simulink library "sm_excv_underc_lib"  (R2023b)
settings: Solver=VariableStepAuto  StartTime=0.0  StopTime=10.0  RelTol=1e-3
undefined symbols (not defined in the file): Excv, L1, L2, L3, L4, L5, L6, L7, L8, L9, P1, P2, P3, P4, P5, P6, P7, P8, P9, shoe_w, X, Y, Z
libraries: sm_tracked_vehicle_lib x70, sm_lib x54, nesl_utility x32, sm_excv_scene_lib x9, fl_lib x8, sm_excv_frame_lib x4
(part 2 of 5)

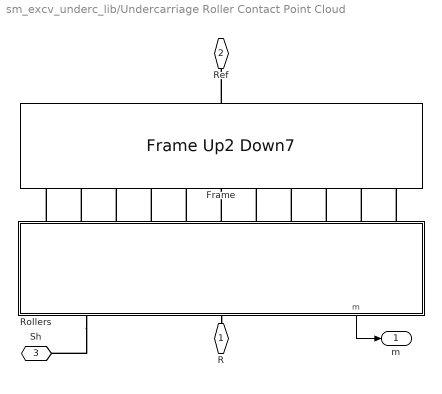
== system sm_excv_underc_lib/Undercarriage Roller Contact Point Cloud ==
  Frame : sm_excv_frame_lib/Frame Up2 Down7  roller_upper_x=roller_upper_x  roller_lower_x=roller_lower_x  idler_x=idler_x  roller_upper_y=roller_upper_y  sprk_pitch_rad=sprk_pitch_rad  roller_lower_rad=roller_lower_rad  plate_h=plate_h  idler_rad=idler_rad  idler_lower_roller_offset_y=idler_lower_roller_offset_y
  Rollers : Subsystem  mask(Rollers with Ground Contact (Point Cloud)){sprk_xc=sprk_xc, sprk_len=sprk_len, sprk_rho=sprk_rho, sprk_clr=sprk_clr, sprk_opc=sprk_opc, sprk_contact_geo_ptcld=sprk_contact_geo_ptcld, sprk_contact_geo_rad=sprk_contact_geo_rad, sprk_contact_geo_clr=sprk_contact_geo_clr, sprk_contact_geo_opc=sprk_contact_geo_opc, idler_rad=idler_rad, idler_len=idler_len, idler_rho=idler_rho, idler_clr=idler_clr, idler_opc=idler_opc, idler_contact_geo_ptcld=idler_contact_geo_ptcld, idler_contact_geo_rad=idler_contact_geo_rad, idler_contact_geo_clr=idler_contact_geo_clr, idler_contact_geo_opc=idler_contact_geo_opc, roller_upper_len=roller_upper_len, roller_upper_rad=roller_upper_rad, roller_upper_rho=roller_upper_rho, roller_upper_clr=roller_upper_clr, roller_upper_opc=roller_upper_opc, roller_upper_contgeo_clr=roller_upper_contgeo_clr, roller_upper_contgeo_opc=roller_upper_contgeo_opc, roller_lower_len=roller_lower_len, roller_lower_rad=roller_lower_rad, roller_lower_rho=roller_lower_rho, roller_lower_clr=roller_lower_clr, roller_lower_opc=roller_lower_opc, roller_lower_contgeo_ptcld=roller_lower_contgeo_ptcld, roller_lower_contgeo_rad=roller_lower_contgeo_rad, roller_lower_contgeo_clr=roller_lower_contgeo_clr, roller_lower_contgeo_opc=roller_lower_contgeo_opc, tensioner_cyl_rad=tensioner_cyl_rad, tensioner_cyl_len=tensioner_cyl_len, tensioner_cyl_rho=tensioner_cyl_rho, tensioner_cyl_clr=tensioner_cyl_clr, tensioner_cyl_opc=tensioner_cyl_opc, tensioner_pist_rad=tensioner_pist_rad, tensioner_pist_len=tensioner_pist_len, tensioner_pist_rho=tensioner_pist_rho, tensioner_pist_clr=tensioner_pist_clr, tensioner_pist_opc=tensioner_pist_opc, tensioner_br_length=tensioner_br_length, tensioner_br_width=tensioner_br_width, tensioner_br_height=tensioner_br_height, tensioner_br_thk=tensioner_br_thk, tensioner_br_rho=tensioner_br_rho, tensioner_br_clr=tensioner_br_clr, tensioner_br_opc=tensioner_br_opc, idler_max_ext=idler_max_ext, sprk_rolling_rad=sprk_rolling_rad, idler_rolling_rad=idler_rolling_rad, roller_lower_rolling_rad=roller_lower_rolling_rad, cyl_len=cyl_len, lext=lext, roller_cyl_clr=roller_cyl_clr, roller_cyl_opc=roller_cyl_opc, sprocket_cyl_clr=sprocket_cyl_clr, sprocket_cyl_opc=sprocket_cyl_opc, idler_cyl_clr=idler_cyl_clr, idler_cyl_opc=idler_cyl_opc, accMx=accMx, accMn=accMn, acc_clr=acc_clr, acc_opc=acc_opc, popup_sense_roller=Actuator Torque}
      mask prompts: sprk_xc "Extrusion Data [x y] (m)"; sprk_len "Length (m)"; sprk_rho "Density (kg/m^3)"; sprk_clr "Color [R G B] (0-1)"; sprk_opc "Opacity (0-1)"; sprk_contact_geo_ptcld "Point Cloud Data [x y z] (m)"; sprk_contact_geo_rad "Point Radius (m)"; sprk_contact_geo_clr "Color [R G B] (0-1)"; sprk_contact_geo_opc "Opacity (0-1)"; idler_rad "Radius (m)"; idler_len "Length(m)"; idler_rho "Density (kg/m^3)"; idler_clr "Color [R G B] (0-1)"; idler_opc "Opacity (0-1)"; idler_contact_geo_ptcld "Point Cloud Data [x y z] (m)"; idler_contact_geo_rad "Point Radius (m)"; idler_contact_geo_clr "Color [R G B] (0-1)"; idler_contact_geo_opc "Opacity (0-1)"; roller_upper_len "Length (m)"; roller_upper_rad "Radius (m)"; roller_upper_rho "Density (kg/m^3)"; roller_upper_clr "Color [R G B] (0-1)"; roller_upper_opc "Opacity (0-1)"; roller_upper_contgeo_clr "Color [R G B] (0-1)"; roller_upper_contgeo_opc "Opacity (0-1)"; roller_lower_len "Length (m)"; roller_lower_rad "Radius (m)"; roller_lower_rho "Density (kg/m^3)"; roller_lower_clr "Color [R G B] (0-1)"; roller_lower_opc "Opacity (0-1)"; roller_lower_contgeo_ptcld "Point Cloud [x y z] (m)"; roller_lower_contgeo_rad "Point Radius (m)"; roller_lower_contgeo_clr "Color [R G B] (0-1)"; roller_lower_contgeo_opc "Opacity (0-1)"; tensioner_cyl_rad "Radius (m)"; tensioner_cyl_len "Length (m)"; tensioner_cyl_rho "Density (kg/m^3)"; tensioner_cyl_clr "Color [R G B] (0-1)"; tensioner_cyl_opc "Opacity (0-1)"; tensioner_pist_rad "Radius (m)"; tensioner_pist_len "Length (m)"; tensioner_pist_rho "Density (kg/m^3)"; tensioner_pist_clr "Color [R G B] (0-1)"; tensioner_pist_opc "Opacity (0.1)"; tensioner_br_length "Length (m)"; tensioner_br_width "Width (m)"; tensioner_br_height "Height (m)"; tensioner_br_thk "Thickness (m)"; tensioner_br_rho "Density (kg/m^3)"; tensioner_br_clr "Color [R G B] (0-1)"; tensioner_br_opc "Opacity (0.1)"; idler_max_ext "Max Extension in Track (m)"; sprk_rolling_rad "Sprocket Rolling Radius (m)"; idler_rolling_rad "Idler Rolling Radius (m)"; roller_lower_rolling_rad "Lower Roller Rolling Radius (m)"; cyl_len "Track Width (m)"; lext "Length Extensions (m)"; roller_cyl_clr "Cylinder Color [R G B] (0-1)"; roller_cyl_opc "Cylinder Opacity (0-1)"; sprocket_cyl_clr "Cylinder Color [R G B] (0-1)"; sprocket_cyl_opc "Cylinder Opacity (0-1)"; idler_cyl_clr "Cylinder Color [R G B] (0-1)"; idler_cyl_opc "Cylinder Opacity (0-1)"; accMx "Accent Max Radius (0-1)"; accMn "Accent Min Radius (0-1)"; acc_clr "Accent Color [R G B] (0-1)"; acc_opc "Accent Opacity (0-1)"; popup_sense_roller "Roller"
      mask help: Models sprocket, rollers, and idler. Components have point cloud contact geometry to enable undercarriage to roll along uneven ground. The sprocket has a 1D rotational mechanical interface to the drivetrain.
      mask init:
      | % Sensing a constraint force can be computationally expensive
      | % Use popup to turn it off if quantity is not needed
      | 
      | if(strcmp(get_param(gcb,'popup_sense_roller'),'Constraint Force'))
      |     set_param([gcb '/Revolute Lower 1'],'SenseConstraintForce','on','SenseTorqueForce','off')
      |     set_param([gcb '/Revolute Lower 2'],'SenseConstraintForce','on','SenseTorqueForce','off')
      |     set_param([gcb '/Revolute Lower 3'],'SenseConstraintForce','on','SenseTorqueForce','off')
      |     set_param([gcb '/Revolute Lower 4'],'SenseConstraintForce','on','SenseTorqueForce','off')
      |     set_param([gcb '/Revolute Lower 5'],'SenseConstraintForce','on','SenseTorqueForce','off')
      |     set_param([gcb '/Revolute Lower 6'],'SenseConstraintForce','on','SenseTorqueForce','off')
      |     set_param([gcb '/Revolute Lower 7'],'SenseConstraintForce','on','SenseTorqueForce','off')
      | else
      |     set_param([gcb '/Revolute Lower 1'],'SenseConstraintForce','off','SenseTorqueForce','on')
      |     set_param([gcb '/Revolute Lower 2'],'SenseConstraintForce','off','SenseTorqueForce','on')
      |     set_param([gcb '/Revolute Lower 3'],'SenseConstraintForce','off','SenseTorqueForce','on')
      |     set_param([gcb '/Revolute Lower 4'],'SenseConstraintForce','off','SenseTorqueForce','on')
      |     set_param([gcb '/Revolute Lower 5'],'SenseConstraintForce','off','SenseTorqueForce','on')
      |     set_param([gcb '/Revolute Lower 6'],'SenseConstraintForce','off','SenseTorqueForce','on')
      |     set_param([gcb '/Revolute Lower 7'],'SenseConstraintForce','off','SenseTorqueForce','on')
      | end
      mask TypeOptions sprk_xc: Sprocket/sprk_xc
      mask TypeOptions sprk_len: Sprocket/sprk_len
      mask TypeOptions sprk_rho: Sprocket/sprk_rho
      mask TypeOptions sprk_clr: Sprocket/sprk_clr
      mask TypeOptions sprk_opc: Sprocket/sprk_opc
      mask TypeOptions sprk_contact_geo_ptcld: Sprocket/sprk_contact_geo_ptcld
      mask TypeOptions sprk_contact_geo_rad: Sprocket/sprk_contact_geo_rad
      mask TypeOptions sprk_contact_geo_clr: Sprocket/sprk_contact_geo_clr
      mask TypeOptions sprk_contact_geo_opc: Sprocket/sprk_contact_geo_opc
      mask TypeOptions idler_rad: Idler/idler_rad
      mask TypeOptions idler_len: Idler/idler_len
      mask TypeOptions idler_rho: Idler/idler_rho
      mask TypeOptions idler_clr: Idler/idler_clr
      mask TypeOptions idler_opc: Idler/idler_opc
      mask TypeOptions idler_contact_geo_ptcld: Idler/idler_contact_geo_ptcld
      mask TypeOptions idler_contact_geo_rad: Idler/idler_contact_geo_rad
      mask TypeOptions idler_contact_geo_clr: Idler/idler_contact_geo_clr
      mask TypeOptions idler_contact_geo_opc: Idler/idler_contact_geo_opc
      mask TypeOptions roller_upper_len:
      | Roller
      | Upper 1/roller_upper_len | Roller
      | Upper 2/roller_upper_len
      mask TypeOptions roller_upper_rad:
      | Roller
      | Upper 1/roller_upper_rad | Roller
      | Upper 2/roller_upper_rad
      mask TypeOptions roller_upper_rho:
      | Roller
      | Upper 1/roller_upper_rho | Roller
      | Upper 2/roller_upper_rho
      mask TypeOptions roller_upper_clr:
      | Roller
      | Upper 1/roller_upper_clr | Roller
      | Upper 2/roller_upper_clr
      mask TypeOptions roller_upper_opc:
      | Roller
      | Upper 1/roller_upper_opc | Roller
      | Upper 2/roller_upper_opc
      mask TypeOptions roller_upper_contgeo_clr:
      | Roller
      | Upper 1/roller_upper_contgeo_clr | Roller
      | Upper 2/roller_upper_contgeo_clr
      mask TypeOptions roller_upper_contgeo_opc:
      | Roller
      | Upper 1/roller_upper_contgeo_opc | Roller
      | Upper 2/roller_upper_contgeo_opc
      mask TypeOptions roller_lower_len:
      | Roller
      | Lower 1/roller_lower_len | Roller
      | Lower 2/roller_lower_len | Roller
      | Lower 3/roller_lower_len | Roller
      | Lower 4/roller_lower_len | Roller
      | Lower 5/roller_lower_len | Roller
      | Lower 6/roller_lower_len | Roller
      | Lower 7/roller_lower_len
      mask TypeOptions roller_lower_rad:
      | Roller
      | Lower 1/roller_lower_rad | Roller
      | Lower 2/roller_lower_rad | Roller
      | Lower 3/roller_lower_rad | Roller
      | Lower 4/roller_lower_rad | Roller
      | Lower 5/roller_lower_rad | Roller
      | Lower 6/roller_lower_rad | Roller
      | Lower 7/roller_lower_rad
      mask TypeOptions roller_lower_rho:
      | Roller
      | Lower 1/roller_lower_rho | Roller
      | Lower 2/roller_lower_rho | Roller
      | Lower 3/roller_lower_rho | Roller
      | Lower 4/roller_lower_rho | Roller
      | Lower 5/roller_lower_rho | Roller
      | Lower 6/roller_lower_rho | Roller
      | Lower 7/roller_lower_rho
      mask TypeOptions roller_lower_clr:
      | Roller
      | Lower 1/roller_lower_clr | Roller
      | Lower 2/roller_lower_clr | Roller
      | Lower 3/roller_lower_clr | Roller
      | Lower 4/roller_lower_clr | Roller
      | Lower 5/roller_lower_clr | Roller
      | Lower 6/roller_lower_clr | Roller
      | Lower 7/roller_lower_clr
      mask TypeOptions roller_lower_opc:
      | Roller
      | Lower 1/roller_lower_opc | Roller
      | Lower 2/roller_lower_opc | Roller
      | Lower 3/roller_lower_opc | Roller
      | Lower 4/roller_lower_opc | Roller
      | Lower 5/roller_lower_opc | Roller
      | Lower 6/roller_lower_opc | Roller
      | Lower 7/roller_lower_opc
      mask TypeOptions roller_lower_contgeo_ptcld:
      | Roller
      | Lower 1/roller_lower_contgeo_ptcld | Roller
      | Lower 2/roller_lower_contgeo_ptcld | Roller
      | Lower 3/roller_lower_contgeo_ptcld | Roller
      | Lower 4/roller_lower_contgeo_ptcld | Roller
      | Lower 5/roller_lower_contgeo_ptcld | Roller
      | Lower 6/roller_lower_contgeo_ptcld | Roller
      | Lower 7/roller_lower_contgeo_ptcld
      mask TypeOptions roller_lower_contgeo_rad:
      | Roller
      | Lower 1/roller_lower_contgeo_rad | Roller
      | Lower 2/roller_lower_contgeo_rad | Roller
      | Lower 3/roller_lower_contgeo_rad | Roller
      | Lower 4/roller_lower_contgeo_rad | Roller
      | Lower 5/roller_lower_contgeo_rad | Roller
      | Lower 6/roller_lower_contgeo_rad | Roller
      | Lower 7/roller_lower_contgeo_rad
      mask TypeOptions roller_lower_contgeo_clr:
      | Roller
      | Lower 1/roller_lower_contgeo_clr | Roller
      | Lower 2/roller_lower_contgeo_clr | Roller
      | Lower 3/roller_lower_contgeo_clr | Roller
      | Lower 4/roller_lower_contgeo_clr | Roller
      | Lower 5/roller_lower_contgeo_clr | Roller
      | Lower 6/roller_lower_contgeo_clr | Roller
      | Lower 7/roller_lower_contgeo_clr
      mask TypeOptions roller_lower_contgeo_opc:
      | Roller
      | Lower 1/roller_lower_contgeo_opc | Roller
      | Lower 2/roller_lower_contgeo_opc | Roller
      | Lower 3/roller_lower_contgeo_opc | Roller
      | Lower 4/roller_lower_contgeo_opc | Roller
      | Lower 5/roller_lower_contgeo_opc | Roller
      | Lower 6/roller_lower_contgeo_opc | Roller
      | Lower 7/roller_lower_contgeo_opc
      mask TypeOptions tensioner_cyl_rad:
      | Tensioner
      | Cylinder/cyl_rad
      mask TypeOptions tensioner_cyl_len:
      | Tensioner
      | Cylinder/cyl_len
      mask TypeOptions tensioner_cyl_rho:
      | Tensioner
      | Cylinder/cyl_rho
      mask TypeOptions tensioner_cyl_clr:
      | Tensioner
      | Cylinder/cyl_clr
      mask TypeOptions tensioner_cyl_opc:
      | Tensioner
      | Cylinder/cyl_opc
      mask TypeOptions tensioner_pist_rad:
      | Tensioner
      | Piston/pist_rad
      mask TypeOptions tensioner_pist_len:
      | Tensioner
      | Piston/pist_len
      mask TypeOptions tensioner_pist_rho:
      | Tensioner
      | Piston/pist_rho
      mask TypeOptions tensioner_pist_clr:
      | Tensioner
      | Piston/pist_clr
      mask TypeOptions tensioner_pist_opc:
      | Tensioner
      | Piston/pist_opc
      mask TypeOptions tensioner_br_length:
      | Tensioner
      | Piston/br_length
      mask TypeOptions tensioner_br_width:
      | Tensioner
      | Piston/br_width
      mask TypeOptions tensioner_br_height:
      | Tensioner
      | Piston/br_height
      mask TypeOptions tensioner_br_thk:
      | Tensioner
      | Piston/br_thk
      mask TypeOptions tensioner_br_rho:
      | Tensioner
      | Piston/br_rho
      mask TypeOptions tensioner_br_clr:
      | Tensioner
      | Piston/br_clr
      mask TypeOptions tensioner_br_opc:
      | Tensioner
      | Piston/br_opc
      mask TypeOptions idler_max_ext:
      | Transform
      | Idler Extend/TranslationStandardOffset
      mask TypeOptions sprk_rolling_rad:
      | Constrain
      | Rollers
      | Idler/sprk_rolling_rad | Sprocket/cyl_rad
      mask TypeOptions idler_rolling_rad:
      | Constrain
      | Rollers
      | Idler/idler_rolling_rad | Idler/cyl_rad
      mask TypeOptions roller_lower_rolling_rad:
      | Constrain
      | Rollers
      | Idler/roller_lower_rolling_rad | Roller
      | Lower 1/cyl_rad | Roller
      | Lower 2/cyl_rad | Roller
      | Lower 3/cyl_rad | Roller
      | Lower 4/cyl_rad | Roller
      | Lower 5/cyl_rad | Roller
      | Lower 6/cyl_rad | Roller
      | Lower 7/cyl_rad
      mask TypeOptions cyl_len:
      | Idler/cyl_len | Roller
      | Lower 1/cyl_len | Roller
      | Lower 2/cyl_len | Roller
      | Lower 3/cyl_len | Roller
      | Lower 4/cyl_len | Roller
      | Lower 5/cyl_len | Roller
      | Lower 6/cyl_len | Roller
      | Lower 7/cyl_len | Sprocket/cyl_len
      mask TypeOptions lext:
      | Idler/lext | Roller
      | Lower 1/lext | Roller
      | Lower 2/lext | Roller
      | Lower 3/lext | Roller
      | Lower 4/lext | Roller
      | Lower 5/lext | Roller
      | Lower 6/lext | Roller
      | Lower 7/lext | Sprocket/lext
      mask TypeOptions roller_cyl_clr:
      | Roller
      | Lower 1/cyl_clr | Roller
      | Lower 2/cyl_clr | Roller
      | Lower 3/cyl_clr | Roller
      | Lower 4/cyl_clr | Roller
      | Lower 5/cyl_clr | Roller
      | Lower 6/cyl_clr | Roller
      | Lower 7/cyl_clr
      mask TypeOptions roller_cyl_opc:
      | Roller
      | Lower 1/cyl_opc | Roller
      | Lower 2/cyl_opc | Roller
      | Lower 3/cyl_opc | Roller
      | Lower 4/cyl_opc | Roller
      | Lower 5/cyl_opc | Roller
      | Lower 6/cyl_opc | Roller
      | Lower 7/cyl_opc
      mask TypeOptions sprocket_cyl_clr: Sprocket/cyl_clr
      mask TypeOptions sprocket_cyl_opc: Sprocket/cyl_opc
      mask TypeOptions idler_cyl_clr: Idler/cyl_clr
      mask TypeOptions idler_cyl_opc: Idler/cyl_opc
      mask TypeOptions accMx:
      | Idler/accMx | Roller
      | Lower 1/accMx | Roller
      | Lower 2/accMx | Roller
      | Lower 3/accMx | Roller
      | Lower 4/accMx | Roller
      | Lower 5/accMx | Roller
      | Lower 6/accMx | Roller
      | Lower 7/accMx | Sprocket/accMx
      mask TypeOptions accMn:
      | Idler/accMn | Roller
      | Lower 1/accMn | Roller
      | Lower 2/accMn | Roller
      | Lower 3/accMn | Roller
      | Lower 4/accMn | Roller
      | Lower 5/accMn | Roller
      | Lower 6/accMn | Roller
      | Lower 7/accMn | Sprocket/accMn
      mask TypeOptions acc_clr:
      | Idler/acc_clr | Roller
      | Lower 1/acc_clr | Roller
      | Lower 2/acc_clr | Roller
      | Lower 3/acc_clr | Roller
      | Lower 4/acc_clr | Roller
      | Lower 5/acc_clr | Roller
      | Lower 6/acc_clr | Roller
      | Lower 7/acc_clr | Sprocket/acc_clr
      mask TypeOptions acc_opc:
      | Idler/acc_opc | Roller
      | Lower 1/acc_opc | Roller
      | Lower 2/acc_opc | Roller
      | Lower 3/acc_opc | Roller
      | Lower 4/acc_opc | Roller
      | Lower 5/acc_opc | Roller
      | Lower 6/acc_opc | Roller
      | Lower 7/acc_opc | Sprocket/acc_opc
      mask TypeOptions popup_sense_roller: Constraint Force | Actuator Torque
      mask DialogControl cont_sprk Prompt: Sprocket
      mask DialogControl cont_sprk_solid Prompt: Solid
      mask DialogControl cont_sprk_contact_geo Prompt: Contact Geometry
      mask DialogControl cont_idler Prompt: Idler
      mask DialogControl cont_idler_solid Prompt: Solid
      mask DialogControl cont_idler_contact_geo Prompt: Contact Geometry
      mask DialogControl cont_rollers Prompt: Rollers
      mask DialogControl cont_roller_upper Prompt: Upper
      mask DialogControl cont_roller_upper_contact_geo Prompt: Contact Geometry
      mask DialogControl cont_lower Prompt: Lower
      mask DialogControl cont_lower_contact_geo Prompt: Contact Geometry
      mask DialogControl cont_tensioner Prompt: Tensioner
      mask DialogControl cont_tensioner_cyl Prompt: Cylinder
      mask DialogControl cont_tensioner_pist Prompt: Piston
      mask DialogControl cont_tensioner_brkt Prompt: Bracket
      mask DialogControl cont_tensioner_assy Prompt: Assembly
      mask DialogControl cont_rolling Prompt: Rolling
      mask DialogControl cont_rolling_constraints Prompt: Constraints and Length
      mask DialogControl cont_rollvis_roller Prompt: Roller Visual: Roller
      mask DialogControl cont_rollvis_sprocket Prompt: Roller Visual: Sprocket
      mask DialogControl cont_rollvis_idler Prompt: Roller Visual: Idler
      mask DialogControl cont_rollvis_accent Prompt: Accent Visual
      mask DialogControl cont_sensing Prompt: Sensing
      mask Display: image('sm_excv_track_rollersptcld_IMAGE.png');
  R : PMIOPort  Side=Right
  Ref : PMIOPort  Port=2  Side=Right
  Sh : PMIOPort  Port=3  Side=Right
  m : Outport
  wires:
  Rollers/1(m) -> m/1
  connections:
  Rollers/RConn2 -- Sh/RConn1
  Rollers/LConn2 -- Frame/RConn2
  Rollers/LConn3 -- Frame/RConn3
  Rollers/LConn11 -- Frame/RConn11
  Rollers/LConn1 -- Frame/RConn1
  Rollers/LConn6 -- Frame/RConn6
  Rollers/LConn9 -- Frame/RConn9
  Rollers/LConn10 -- Frame/RConn10
  Rollers/LConn8 -- Frame/RConn8
  Rollers/LConn4 -- Frame/RConn4
  Rollers/LConn5 -- Frame/RConn5
  Rollers/LConn7 -- Frame/RConn7
  Frame/LConn1 -- Ref/RConn1
  Rollers/RConn1 -- R/RConn1

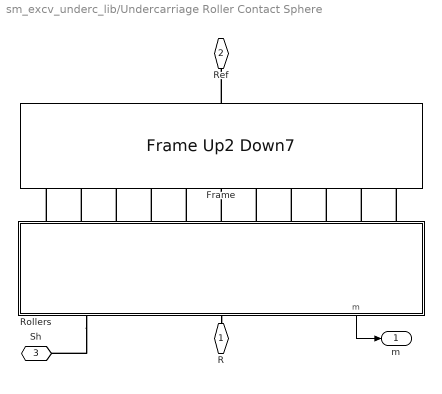
== system sm_excv_underc_lib/Undercarriage Roller Contact Sphere ==
  Frame : sm_excv_frame_lib/Frame Up2 Down7  roller_upper_x=roller_upper_x  roller_lower_x=roller_lower_x  idler_x=idler_x  roller_upper_y=roller_upper_y  sprk_pitch_rad=sprk_pitch_rad  roller_lower_rad=roller_lower_rad  plate_h=plate_h  idler_rad=idler_rad  idler_lower_roller_offset_y=idler_lower_roller_offset_y
  Rollers : Subsystem  mask(Rollers with Ground Contact (Spheres)){sprk_xc=sprk_xc, sprk_len=sprk_len, sprk_rho=sprk_rho, sprk_clr=sprk_clr, sprk_opc=sprk_opc, sprk_contact_geo_clr=sprk_contact_geo_clr, sprk_contact_geo_opc=sprk_contact_geo_opc, idler_rad=idler_rad, idler_len=idler_len, idler_rho=idler_rho, idler_clr=idler_clr, idler_opc=idler_opc, idler_contact_geo_clr=idler_contact_geo_clr, idler_contact_geo_opc=idler_contact_geo_opc, roller_upper_len=roller_upper_len, roller_upper_rad=roller_upper_rad, roller_upper_rho=roller_upper_rho, roller_upper_clr=roller_upper_clr, roller_upper_opc=roller_upper_opc, roller_upper_contgeo_clr=roller_upper_contgeo_clr, roller_upper_contgeo_opc=roller_upper_contgeo_opc, roller_lower_len=roller_lower_len, roller_lower_rad=roller_lower_rad, roller_lower_rho=roller_lower_rho, roller_lower_clr=roller_lower_clr, roller_lower_opc=roller_lower_opc, roller_lower_contgeo_clr=roller_lower_contgeo_clr, roller_lower_contgeo_opc=roller_lower_contgeo_opc, tensioner_cyl_rad=tensioner_cyl_rad, tensioner_cyl_len=tensioner_cyl_len, tensioner_cyl_rho=tensioner_cyl_rho, tensioner_cyl_clr=tensioner_cyl_clr, tensioner_cyl_opc=tensioner_cyl_opc, tensioner_pist_rad=tensioner_pist_rad, tensioner_pist_len=tensioner_pist_len, tensioner_pist_rho=tensioner_pist_rho, tensioner_pist_clr=tensioner_pist_clr, tensioner_pist_opc=tensioner_pist_opc, tensioner_br_length=tensioner_br_length, tensioner_br_width=tensioner_br_width, tensioner_br_height=tensioner_br_height, tensioner_br_thk=tensioner_br_thk, tensioner_br_rho=tensioner_br_rho, tensioner_br_clr=tensioner_br_clr, tensioner_br_opc=tensioner_br_opc, idler_max_ext=idler_max_ext, sprk_rolling_rad=sprk_rolling_rad, idler_rolling_rad=idler_rolling_rad, roller_lower_rolling_rad=roller_lower_rolling_rad, shoe_w=shoe_w, popup_sense_roller=Actuator Torque}
      mask prompts: sprk_xc "Extrusion Data [x y] (m)"; sprk_len "Length (m)"; sprk_rho "Density (kg/m^3)"; sprk_clr "Color [R G B] (0-1)"; sprk_opc "Opacity (0-1)"; sprk_contact_geo_clr "Color [R G B] (0-1)"; sprk_contact_geo_opc "Opacity (0-1)"; idler_rad "Radius (m)"; idler_len "Length(m)"; idler_rho "Density (kg/m^3)"; idler_clr "Color [R G B] (0-1)"; idler_opc "Opacity (0-1)"; idler_contact_geo_clr "Color [R G B] (0-1)"; idler_contact_geo_opc "Opacity (0-1)"; roller_upper_len "Length (m)"; roller_upper_rad "Radius (m)"; roller_upper_rho "Density (kg/m^3)"; roller_upper_clr "Color [R G B] (0-1)"; roller_upper_opc "Opacity (0-1)"; roller_upper_contgeo_clr "Color [R G B] (0-1)"; roller_upper_contgeo_opc "Opacity (0-1)"; roller_lower_len "Length (m)"; roller_lower_rad "Radius (m)"; roller_lower_rho "Density (kg/m^3)"; roller_lower_clr "Color [R G B] (0-1)"; roller_lower_opc "Opacity (0-1)"; roller_lower_contgeo_clr "Color [R G B] (0-1)"; roller_lower_contgeo_opc "Opacity (0-1)"; tensioner_cyl_rad "Radius (m)"; tensioner_cyl_len "Length (m)"; tensioner_cyl_rho "Density (kg/m^3)"; tensioner_cyl_clr "Color [R G B] (0-1)"; tensioner_cyl_opc "Opacity (0-1)"; tensioner_pist_rad "Radius (m)"; tensioner_pist_len "Length (m)"; tensioner_pist_rho "Density (kg/m^3)"; tensioner_pist_clr "Color [R G B] (0-1)"; tensioner_pist_opc "Opacity (0.1)"; tensioner_br_length "Length (m)"; tensioner_br_width "Width (m)"; tensioner_br_height "Height (m)"; tensioner_br_thk "Thickness (m)"; tensioner_br_rho "Density (kg/m^3)"; tensioner_br_clr "Color [R G B] (0-1)"; tensioner_br_opc "Opacity (0.1)"; idler_max_ext "Max Extension in Track (m)"; sprk_rolling_rad "Sprocket Rolling Radius (m)"; idler_rolling_rad "Idler Rolling Radius (m)"; roller_lower_rolling_rad "Lower Roller Rolling Radius (m)"; shoe_w "Shoe Width (m)"; popup_sense_roller "Roller"
      mask help: Models sprocket, rollers, and idler. Components have sphere contact geometry to enable undercarriage to roll along uneven ground. The sprocket has a 1D rotational mechanical interface to the drivetrain.
      mask init:
      | % Sensing a constraint force can be computationally expensive
      | % Use popup to turn it off if quantity is not needed
      | if(popup_sense_roller == 1)
      |     set_param([gcb '/Revolute Lower 1'],'SenseConstraintForce','on','SenseTorqueForce','off')
      |     set_param([gcb '/Revolute Lower 2'],'SenseConstraintForce','on','SenseTorqueForce','off')
      |     set_param([gcb '/Revolute Lower 3'],'SenseConstraintForce','on','SenseTorqueForce','off')
      |     set_param([gcb '/Revolute Lower 4'],'SenseConstraintForce','on','SenseTorqueForce','off')
      |     set_param([gcb '/Revolute Lower 5'],'SenseConstraintForce','on','SenseTorqueForce','off')
      |     set_param([gcb '/Revolute Lower 6'],'SenseConstraintForce','on','SenseTorqueForce','off')
      |     set_param([gcb '/Revolute Lower 7'],'SenseConstraintForce','on','SenseTorqueForce','off')
      | else
      |     set_param([gcb '/Revolute Lower 1'],'SenseConstraintForce','off','SenseTorqueForce','on')
      |     set_param([gcb '/Revolute Lower 2'],'SenseConstraintForce','off','SenseTorqueForce','on')
      |     set_param([gcb '/Revolute Lower 3'],'SenseConstraintForce','off','SenseTorqueForce','on')
      |     set_param([gcb '/Revolute Lower 4'],'SenseConstraintForce','off','SenseTorqueForce','on')
      |     set_param([gcb '/Revolute Lower 5'],'SenseConstraintForce','off','SenseTorqueForce','on')
      |     set_param([gcb '/Revolute Lower 6'],'SenseConstraintForce','off','SenseTorqueForce','on')
      |     set_param([gcb '/Revolute Lower 7'],'SenseConstraintForce','off','SenseTorqueForce','on')
      | end
      mask TypeOptions sprk_xc: Sprocket/sprk_xc
      mask TypeOptions sprk_len: Sprocket/sprk_len
      mask TypeOptions sprk_rho: Sprocket/sprk_rho
      mask TypeOptions sprk_clr: Sprocket/sprk_clr
      mask TypeOptions sprk_opc: Sprocket/sprk_opc
      mask TypeOptions sprk_contact_geo_clr: Sprocket/sprk_contact_geo_clr
      mask TypeOptions sprk_contact_geo_opc: Sprocket/sprk_contact_geo_opc
      mask TypeOptions idler_rad: Idler/idler_rad
      mask TypeOptions idler_len: Idler/idler_len
      mask TypeOptions idler_rho: Idler/idler_rho
      mask TypeOptions idler_clr: Idler/idler_clr
      mask TypeOptions idler_opc: Idler/idler_opc
      mask TypeOptions idler_contact_geo_clr: Idler/idler_contact_geo_clr
      mask TypeOptions idler_contact_geo_opc: Idler/idler_contact_geo_opc
      mask TypeOptions roller_upper_len:
      | Roller
      | Upper 1/roller_upper_len | Roller
      | Upper 2/roller_upper_len
      mask TypeOptions roller_upper_rad:
      | Roller
      | Upper 1/roller_upper_rad | Roller
      | Upper 2/roller_upper_rad
      mask TypeOptions roller_upper_rho:
      | Roller
      | Upper 1/roller_upper_rho | Roller
      | Upper 2/roller_upper_rho
      mask TypeOptions roller_upper_clr:
      | Roller
      | Upper 1/roller_upper_clr | Roller
      | Upper 2/roller_upper_clr
      mask TypeOptions roller_upper_opc:
      | Roller
      | Upper 1/roller_upper_opc | Roller
      | Upper 2/roller_upper_opc
      mask TypeOptions roller_upper_contgeo_clr:
      | Roller
      | Upper 1/roller_upper_contgeo_clr | Roller
      | Upper 2/roller_upper_contgeo_clr
      mask TypeOptions roller_upper_contgeo_opc:
      | Roller
      | Upper 1/roller_upper_contgeo_opc | Roller
      | Upper 2/roller_upper_contgeo_opc
      mask TypeOptions roller_lower_len:
      | Roller
      | Lower 1/roller_lower_len | Roller
      | Lower 2/roller_lower_len | Roller
      | Lower 3/roller_lower_len | Roller
      | Lower 4/roller_lower_len | Roller
      | Lower 5/roller_lower_len | Roller
      | Lower 6/roller_lower_len | Roller
      | Lower 7/roller_lower_len
      mask TypeOptions roller_lower_rad:
      | Roller
      | Lower 1/roller_lower_rad | Roller
      | Lower 2/roller_lower_rad | Roller
      | Lower 3/roller_lower_rad | Roller
      | Lower 4/roller_lower_rad | Roller
      | Lower 5/roller_lower_rad | Roller
      | Lower 6/roller_lower_rad | Roller
      | Lower 7/roller_lower_rad
      mask TypeOptions roller_lower_rho:
      | Roller
      | Lower 1/roller_lower_rho | Roller
      | Lower 2/roller_lower_rho | Roller
      | Lower 3/roller_lower_rho | Roller
      | Lower 4/roller_lower_rho | Roller
      | Lower 5/roller_lower_rho | Roller
      | Lower 6/roller_lower_rho | Roller
      | Lower 7/roller_lower_rho
      mask TypeOptions roller_lower_clr:
      | Roller
      | Lower 1/roller_lower_clr | Roller
      | Lower 2/roller_lower_clr | Roller
      | Lower 3/roller_lower_clr | Roller
      | Lower 4/roller_lower_clr | Roller
      | Lower 5/roller_lower_clr | Roller
      | Lower 6/roller_lower_clr | Roller
      | Lower 7/roller_lower_clr
      mask TypeOptions roller_lower_opc:
      | Roller
      | Lower 1/roller_lower_opc | Roller
      | Lower 2/roller_lower_opc | Roller
      | Lower 3/roller_lower_opc | Roller
      | Lower 4/roller_lower_opc | Roller
      | Lower 5/roller_lower_opc | Roller
      | Lower 6/roller_lower_opc | Roller
      | Lower 7/roller_lower_opc
      mask TypeOptions roller_lower_contgeo_clr:
      | Roller
      | Lower 1/roller_lower_contgeo_clr | Roller
      | Lower 2/roller_lower_contgeo_clr | Roller
      | Lower 3/roller_lower_contgeo_clr | Roller
      | Lower 4/roller_lower_contgeo_clr | Roller
      | Lower 5/roller_lower_contgeo_clr | Roller
      | Lower 6/roller_lower_contgeo_clr | Roller
      | Lower 7/roller_lower_contgeo_clr
      mask TypeOptions roller_lower_contgeo_opc:
      | Roller
      | Lower 1/roller_lower_contgeo_opc | Roller
      | Lower 2/roller_lower_contgeo_opc | Roller
      | Lower 3/roller_lower_contgeo_opc | Roller
      | Lower 4/roller_lower_contgeo_opc | Roller
      | Lower 5/roller_lower_contgeo_opc | Roller
      | Lower 6/roller_lower_contgeo_opc | Roller
      | Lower 7/roller_lower_contgeo_opc
      mask TypeOptions tensioner_cyl_rad:
      | Tensioner
      | Cylinder/cyl_rad
      mask TypeOptions tensioner_cyl_len:
      | Tensioner
      | Cylinder/cyl_len
      mask TypeOptions tensioner_cyl_rho:
      | Tensioner
      | Cylinder/cyl_rho
      mask TypeOptions tensioner_cyl_clr:
      | Tensioner
      | Cylinder/cyl_clr
      mask TypeOptions tensioner_cyl_opc:
      | Tensioner
      | Cylinder/cyl_opc
      mask TypeOptions tensioner_pist_rad:
      | Tensioner
      | Piston/pist_rad
      mask TypeOptions tensioner_pist_len:
      | Tensioner
      | Piston/pist_len
      mask TypeOptions tensioner_pist_rho:
      | Tensioner
      | Piston/pist_rho
      mask TypeOptions tensioner_pist_clr:
      | Tensioner
      | Piston/pist_clr
      mask TypeOptions tensioner_pist_opc:
      | Tensioner
      | Piston/pist_opc
      mask TypeOptions tensioner_br_length:
      | Tensioner
      | Piston/br_length
      mask TypeOptions tensioner_br_width:
      | Tensioner
      | Piston/br_width
      mask TypeOptions tensioner_br_height:
      | Tensioner
      | Piston/br_height
      mask TypeOptions tensioner_br_thk:
      | Tensioner
      | Piston/br_thk
      mask TypeOptions tensioner_br_rho:
      | Tensioner
      | Piston/br_rho
      mask TypeOptions tensioner_br_clr:
      | Tensioner
      | Piston/br_clr
      mask TypeOptions tensioner_br_opc:
      | Tensioner
      | Piston/br_opc
      mask TypeOptions idler_max_ext:
      | Transform
      | Idler Extend/TranslationStandardOffset
      mask TypeOptions sprk_rolling_rad:
      | Constrain
      | Rollers
      | Idler/sprk_rolling_rad | Sprocket/sprk_rolling_rad
      mask TypeOptions idler_rolling_rad:
      | Constrain
      | Rollers
      | Idler/idler_rolling_rad | Idler/idler_rolling_rad
      mask TypeOptions roller_lower_rolling_rad:
      | Constrain
      | Rollers
      | Idler/roller_lower_rolling_rad | Roller
      | Lower 1/roller_lower_rolling_rad | Roller
      | Lower 2/roller_lower_rolling_rad | Roller
      | Lower 3/roller_lower_rolling_rad | Roller
      | Lower 4/roller_lower_rolling_rad | Roller
      | Lower 5/roller_lower_rolling_rad | Roller
      | Lower 6/roller_lower_rolling_rad | Roller
      | Lower 7/roller_lower_rolling_rad
      mask TypeOptions shoe_w:
      | Idler/idler_contact_geo_width | Roller
      | Lower 1/roller_lower_contgeo_width | Roller
      | Lower 2/roller_lower_contgeo_width | Roller
      | Lower 3/roller_lower_contgeo_width | Roller
      | Lower 4/roller_lower_contgeo_width | Roller
      | Lower 5/roller_lower_contgeo_width | Roller
      | Lower 6/roller_lower_contgeo_width | Roller
      | Lower 7/roller_lower_contgeo_width | Sprocket/sprk_contact_geo_w
      mask TypeOptions popup_sense_roller: Constraint Force | Actuator Torque
      mask DialogControl cont_sprk Prompt: Sprocket
      mask DialogControl cont_sprk_solid Prompt: Solid
      mask DialogControl cont_sprk_contact_geo Prompt: Contact Geometry
      mask DialogControl cont_idler Prompt: Idler
      mask DialogControl cont_idler_solid Prompt: Solid
      mask DialogControl cont_idler_contact_geo Prompt: Contact Geometry
      mask DialogControl cont_rollers Prompt: Rollers
      mask DialogControl cont_roller_upper Prompt: Upper
      mask DialogControl cont_roller_upper_contact_geo Prompt: Contact Geometry
      mask DialogControl cont_lower Prompt: Lower
      mask DialogControl cont_lower_contact_geo Prompt: Contact Geometry
      mask DialogControl cont_tensioner Prompt: Tensioner
      mask DialogControl cont_tensioner_cyl Prompt: Cylinder
      mask DialogControl cont_tensioner_pist Prompt: Piston
      mask DialogControl cont_tensioner_brkt Prompt: Bracket
      mask DialogControl cont_tensioner_assy Prompt: Assembly
      mask DialogControl cont_rolling Prompt: Rolling
      mask DialogControl cont_constr_len Prompt: Constraints and Length
      mask DialogControl cont_sensing Prompt: Sensing
      mask Display: image('sm_excv_track_rollerssphere_IMAGE.png');
  R : PMIOPort  Side=Right
  Ref : PMIOPort  Port=2  Side=Right
  Sh : PMIOPort  Port=3  Side=Right
  m : Outport
  wires:
  Rollers/1(m) -> m/1
  connections:
  Rollers/RConn1 -- R/RConn1
  Frame/LConn1 -- Ref/RConn1
  Rollers/LConn7 -- Frame/RConn7
  Rollers/LConn5 -- Frame/RConn5
  Rollers/LConn4 -- Frame/RConn4
  Rollers/LConn8 -- Frame/RConn8
  Rollers/LConn10 -- Frame/RConn10
  Rollers/LConn9 -- Frame/RConn9
  Rollers/LConn6 -- Frame/RConn6
  Rollers/LConn1 -- Frame/RConn1
  Rollers/LConn11 -- Frame/RConn11
  Rollers/LConn3 -- Frame/RConn3
  Rollers/LConn2 -- Frame/RConn2
  Rollers/RConn2 -- Sh/RConn1

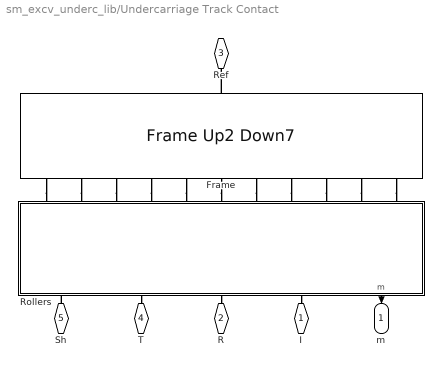
== system sm_excv_underc_lib/Undercarriage Track Contact ==
  Frame : sm_excv_frame_lib/Frame Up2 Down7  roller_upper_x=roller_upper_x  roller_lower_x=roller_lower_x  idler_x=idler_x  roller_upper_y=roller_upper_y  sprk_pitch_rad=sprk_pitch_rad  roller_lower_rad=roller_lower_rad  plate_h=plate_h  idler_rad=idler_rad  idler_lower_roller_offset_y=idler_lower_roller_offset_y
  Rollers : Subsystem  mask(Rollers for Integration with Track Model){sprk_xc=sprk_xc, sprk_len=sprk_len, sprk_rho=sprk_rho, sprk_clr=sprk_clr, sprk_opc=sprk_opc, sprk_contact_geo_ptcld=sprk_contact_geo_ptcld, sprk_contact_geo_rad=sprk_contact_geo_rad, sprk_contact_geo_clr=sprk_contact_geo_clr, sprk_contact_geo_opc=sprk_contact_geo_opc, idler_rad=idler_rad, idler_len=idler_len, idler_rho=idler_rho, idler_clr=idler_clr, idler_opc=idler_opc, idler_contgeo_clr=idler_contgeo_clr, idler_contgeo_opc=idler_contgeo_opc, roller_upper_len=roller_upper_len, roller_upper_rad=roller_upper_rad, roller_upper_rho=roller_upper_rho, roller_upper_clr=roller_upper_clr, roller_upper_opc=roller_upper_opc, roller_upper_contgeo_clr=roller_upper_contgeo_clr, roller_upper_contgeo_opc=roller_upper_contgeo_opc, roller_lower_len=roller_lower_len, roller_lower_rad=roller_lower_rad, roller_lower_rho=roller_lower_rho, roller_lower_clr=roller_lower_clr, roller_lower_opc=roller_lower_opc, roller_lower_contgeo_clr=roller_lower_contgeo_clr, roller_lower_contgeo_opc=roller_lower_contgeo_opc, tensioner_cyl_rad=tensioner_cyl_rad, tensioner_cyl_len=tensioner_cyl_len, tensioner_cyl_rho=tensioner_cyl_rho, tensioner_cyl_clr=tensioner_cyl_clr, tensioner_cyl_opc=tensioner_cyl_opc, tensioner_pist_rad=tensioner_pist_rad, tensioner_pist_len=tensioner_pist_len, tensioner_pist_rho=tensioner_pist_rho, tensioner_pist_clr=tensioner_pist_clr, tensioner_pist_opc=tensioner_pist_opc, tensioner_br_length=tensioner_br_length, tensioner_br_width=tensioner_br_width, tensioner_br_height=tensioner_br_height, tensioner_br_thk=tensioner_br_thk, tensioner_br_rho=tensioner_br_rho, tensioner_br_clr=tensioner_br_clr, tensioner_br_opc=tensioner_br_opc, tensioner_eqpos=tensioner_eqpos, tensioner_x0=tensioner_x0, tensioner_b=tensioner_b, tensioner_k=tensioner_k, popup_sense_roller=Actuator Torque}
      mask prompts: sprk_xc "Extrusion Data [x y] (m)"; sprk_len "Length (m)"; sprk_rho "Density (kg/m^3)"; sprk_clr "Color [R G B] (0-1)"; sprk_opc "Opacity (0-1)"; sprk_contact_geo_ptcld "Point Cloud Data [x y z] (m)"; sprk_contact_geo_rad "Radius (m)"; sprk_contact_geo_clr "Color [R G B] (0-1)"; sprk_contact_geo_opc "Opacity (0-1)"; idler_rad "Radius (m)"; idler_len "Length(m)"; idler_rho "Density (kg/m^3)"; idler_clr "Color [R G B] (0-1)"; idler_opc "Opacity (0-1)"; idler_contgeo_clr "Color [R G B] (0-1)"; idler_contgeo_opc "Opacity (0-1)"; roller_upper_len "Length (m)"; roller_upper_rad "Radius (m)"; roller_upper_rho "Density (kg/m^3)"; roller_upper_clr "Color [R G B] (0-1)"; roller_upper_opc "Opacity (0-1)"; roller_upper_contgeo_clr "Color [R G B] (0-1)"; roller_upper_contgeo_opc "Opacity (0-1)"; roller_lower_len "Length (m)"; roller_lower_rad "Radius (m)"; roller_lower_rho "Density (kg/m^3)"; roller_lower_clr "Color [R G B] (0-1)"; roller_lower_opc "Opacity (0-1)"; roller_lower_contgeo_clr "Color [R G B] (0-1)"; roller_lower_contgeo_opc "Opacity (0-1)"; tensioner_cyl_rad "Radius (m)"; tensioner_cyl_len "Length (m)"; tensioner_cyl_rho "Density (kg/m^3)"; tensioner_cyl_clr "Color [R G B] (0-1)"; tensioner_cyl_opc "Opacity (0-1)"; tensioner_pist_rad "Radius (m)"; tensioner_pist_len "Length (m)"; tensioner_pist_rho "Density (kg/m^3)"; tensioner_pist_clr "Color [R G B] (0-1)"; tensioner_pist_opc "Opacity (0.1)"; tensioner_br_length "Length (m)"; tensioner_br_width "Width (m)"; tensioner_br_height "Height (m)"; tensioner_br_thk "Thickness (m)"; tensioner_br_rho "Density (kg/m^3)"; tensioner_br_clr "Color [R G B] (0-1)"; tensioner_br_opc "Opacity (0.1)"; tensioner_eqpos "Equilibrium Position (m)"; tensioner_x0 "Assembly Position (m)"; tensioner_b "Damping Coefficient (N/(m/s))"; tensioner_k "Stiffness Coefficient (N/m)"; popup_sense_roller "Roller"
      mask help: Models sprocket, rollers, and idler with tensioner. Components have contact geometry for integration with a segmented track model. The sprocket has a 1D rotational mechanical interface to the drivetrain.
      mask init:
      | % Sensing a constraint force can be computationally expensive
      | % Use popup to turn it off if quantity is not needed
      | if(strcmp(get_param(gcb,'popup_sense_roller'),'Constraint Force'))
      |     set_param([gcb '/Revolute Lower 1'],'SenseConstraintForce','on','SenseTorqueForce','off')
      |     set_param([gcb '/Revolute Lower 2'],'SenseConstraintForce','on','SenseTorqueForce','off')
      |     set_param([gcb '/Revolute Lower 3'],'SenseConstraintForce','on','SenseTorqueForce','off')
      |     set_param([gcb '/Revolute Lower 4'],'SenseConstraintForce','on','SenseTorqueForce','off')
      |     set_param([gcb '/Revolute Lower 5'],'SenseConstraintForce','on','SenseTorqueForce','off')
      |     set_param([gcb '/Revolute Lower 6'],'SenseConstraintForce','on','SenseTorqueForce','off')
      |     set_param([gcb '/Revolute Lower 7'],'SenseConstraintForce','on','SenseTorqueForce','off')
      | else
      |     set_param([gcb '/Revolute Lower 1'],'SenseConstraintForce','off','SenseTorqueForce','on')
      |     set_param([gcb '/Revolute Lower 2'],'SenseConstraintForce','off','SenseTorqueForce','on')
      |     set_param([gcb '/Revolute Lower 3'],'SenseConstraintForce','off','SenseTorqueForce','on')
      |     set_param([gcb '/Revolute Lower 4'],'SenseConstraintForce','off','SenseTorqueForce','on')
      |     set_param([gcb '/Revolute Lower 5'],'SenseConstraintForce','off','SenseTorqueForce','on')
      |     set_param([gcb '/Revolute Lower 6'],'SenseConstraintForce','off','SenseTorqueForce','on')
      |     set_param([gcb '/Revolute Lower 7'],'SenseConstraintForce','off','SenseTorqueForce','on')
      | end
      mask TypeOptions sprk_xc: Sprocket/sprk_xc
      mask TypeOptions sprk_len: Sprocket/sprk_len
      mask TypeOptions sprk_rho: Sprocket/sprk_rho
      mask TypeOptions sprk_clr: Sprocket/sprk_clr
      mask TypeOptions sprk_opc: Sprocket/sprk_opc
      mask TypeOptions sprk_contact_geo_ptcld: Sprocket/sprk_contact_geo_ptcld
      mask TypeOptions sprk_contact_geo_rad: Sprocket/sprk_contact_geo_rad
      mask TypeOptions sprk_contact_geo_clr: Sprocket/sprk_contact_geo_clr
      mask TypeOptions sprk_contact_geo_opc: Sprocket/sprk_contact_geo_opc
      mask TypeOptions idler_rad: Idler/idler_rad
      mask TypeOptions idler_len: Idler/idler_len
      mask TypeOptions idler_rho: Idler/idler_rho
      mask TypeOptions idler_clr: Idler/idler_clr
      mask TypeOptions idler_opc: Idler/idler_opc
      mask TypeOptions idler_contgeo_clr: Idler/idler_contgeo_clr
      mask TypeOptions idler_contgeo_opc: Idler/idler_contgeo_opc
      mask TypeOptions roller_upper_len:
      | Roller
      | Upper 1/roller_upper_len | Roller
      | Upper 2/roller_upper_len
      mask TypeOptions roller_upper_rad:
      | Roller
      | Upper 1/roller_upper_rad | Roller
      | Upper 2/roller_upper_rad
      mask TypeOptions roller_upper_rho:
      | Roller
      | Upper 1/roller_upper_rho | Roller
      | Upper 2/roller_upper_rho
      mask TypeOptions roller_upper_clr:
      | Roller
      | Upper 1/roller_upper_clr | Roller
      | Upper 2/roller_upper_clr
      mask TypeOptions roller_upper_opc:
      | Roller
      | Upper 1/roller_upper_opc | Roller
      | Upper 2/roller_upper_opc
      mask TypeOptions roller_upper_contgeo_clr:
      | Roller
      | Upper 1/roller_upper_contgeo_clr | Roller
      | Upper 2/roller_upper_contgeo_clr
      mask TypeOptions roller_upper_contgeo_opc:
      | Roller
      | Upper 1/roller_upper_contgeo_opc | Roller
      | Upper 2/roller_upper_contgeo_opc
      mask TypeOptions roller_lower_len:
      | Roller
      | Lower 1/roller_lower_len | Roller
      | Lower 2/roller_lower_len | Roller
      | Lower 3/roller_lower_len | Roller
      | Lower 4/roller_lower_len | Roller
      | Lower 5/roller_lower_len | Roller
      | Lower 6/roller_lower_len | Roller
      | Lower 7/roller_lower_len
      mask TypeOptions roller_lower_rad:
      | Roller
      | Lower 1/roller_lower_rad | Roller
      | Lower 2/roller_lower_rad | Roller
      | Lower 3/roller_lower_rad | Roller
      | Lower 4/roller_lower_rad | Roller
      | Lower 5/roller_lower_rad | Roller
      | Lower 6/roller_lower_rad | Roller
      | Lower 7/roller_lower_rad
      mask TypeOptions roller_lower_rho:
      | Roller
      | Lower 1/roller_lower_rho | Roller
      | Lower 2/roller_lower_rho | Roller
      | Lower 3/roller_lower_rho | Roller
      | Lower 4/roller_lower_rho | Roller
      | Lower 5/roller_lower_rho | Roller
      | Lower 6/roller_lower_rho | Roller
      | Lower 7/roller_lower_rho
      mask TypeOptions roller_lower_clr:
      | Roller
      | Lower 1/roller_lower_clr | Roller
      | Lower 2/roller_lower_clr | Roller
      | Lower 3/roller_lower_clr | Roller
      | Lower 4/roller_lower_clr | Roller
      | Lower 5/roller_lower_clr | Roller
      | Lower 6/roller_lower_clr | Roller
      | Lower 7/roller_lower_clr
      mask TypeOptions roller_lower_opc:
      | Roller
      | Lower 1/roller_lower_opc | Roller
      | Lower 2/roller_lower_opc | Roller
      | Lower 3/roller_lower_opc | Roller
      | Lower 4/roller_lower_opc | Roller
      | Lower 5/roller_lower_opc | Roller
      | Lower 6/roller_lower_opc | Roller
      | Lower 7/roller_lower_opc
      mask TypeOptions roller_lower_contgeo_clr:
      | Roller
      | Lower 1/roller_lower_contgeo_clr | Roller
      | Lower 2/roller_lower_contgeo_clr | Roller
      | Lower 3/roller_lower_contgeo_clr | Roller
      | Lower 4/roller_lower_contgeo_clr | Roller
      | Lower 5/roller_lower_contgeo_clr | Roller
      | Lower 6/roller_lower_contgeo_clr | Roller
      | Lower 7/roller_lower_contgeo_clr
      mask TypeOptions roller_lower_contgeo_opc:
      | Roller
      | Lower 1/roller_lower_contgeo_opc | Roller
      | Lower 2/roller_lower_contgeo_opc | Roller
      | Lower 3/roller_lower_contgeo_opc | Roller
      | Lower 4/roller_lower_contgeo_opc | Roller
      | Lower 5/roller_lower_contgeo_opc | Roller
      | Lower 6/roller_lower_contgeo_opc | Roller
      | Lower 7/roller_lower_contgeo_opc
      mask TypeOptions tensioner_cyl_rad:
      | Tensioner
      | Cylinder/cyl_rad
      mask TypeOptions tensioner_cyl_len:
      | Tensioner
      | Cylinder/cyl_len
      mask TypeOptions tensioner_cyl_rho:
      | Tensioner
      | Cylinder/cyl_rho
      mask TypeOptions tensioner_cyl_clr:
      | Tensioner
      | Cylinder/cyl_clr
      mask TypeOptions tensioner_cyl_opc:
      | Tensioner
      | Cylinder/cyl_opc
      mask TypeOptions tensioner_pist_rad:
      | Tensioner
      | Piston/pist_rad
      mask TypeOptions tensioner_pist_len:
      | Tensioner
      | Piston/pist_len
      mask TypeOptions tensioner_pist_rho:
      | Tensioner
      | Piston/pist_rho
      mask TypeOptions tensioner_pist_clr:
      | Tensioner
      | Piston/pist_clr
      mask TypeOptions tensioner_pist_opc:
      | Tensioner
      | Piston/pist_opc
      mask TypeOptions tensioner_br_length:
      | Tensioner
      | Piston/br_length
      mask TypeOptions tensioner_br_width:
      | Tensioner
      | Piston/br_width
      mask TypeOptions tensioner_br_height:
      | Tensioner
      | Piston/br_height
      mask TypeOptions tensioner_br_thk:
      | Tensioner
      | Piston/br_thk
      mask TypeOptions tensioner_br_rho:
      | Tensioner
      | Piston/br_rho
      mask TypeOptions tensioner_br_clr:
      | Tensioner
      | Piston/br_clr
      mask TypeOptions tensioner_br_opc:
      | Tensioner
      | Piston/br_opc
      mask TypeOptions tensioner_eqpos:
      | Prismatic
      | Tensioner/EquilibriumPosition
      mask TypeOptions tensioner_x0:
      | Prismatic
      | Tensioner/PositionTargetValue
      mask TypeOptions tensioner_b:
      | Prismatic
      | Tensioner/DampingCoefficient
      mask TypeOptions tensioner_k:
      | Prismatic
      | Tensioner/SpringStiffness
      mask TypeOptions popup_sense_roller: Constraint Force | Actuator Torque
      mask DialogControl cont_sprk Prompt: Sprocket
      mask DialogControl cont_sprk_solid Prompt: Solid
      mask DialogControl cont_sprk_contact_geo Prompt: Contact Geometry
      mask DialogControl cont_idler Prompt: Idler
      mask DialogControl cont_idler_solid Prompt: Solid
      mask DialogControl cont_idler_contact_geo Prompt: Contact Geometry
      mask DialogControl cont_rollers Prompt: Rollers
      mask DialogControl cont_roller_upper Prompt: Upper
      mask DialogControl cont_roller_upper_contact_geo Prompt: Contact Geometry
      mask DialogControl cont_lower Prompt: Lower
      mask DialogControl cont_lower_contact_geo Prompt: Contact Geometry
      mask DialogControl cont_tensioner Prompt: Tensioner
      mask DialogControl cont_tensioner_cyl Prompt: Cylinder
      mask DialogControl cont_tensioner_pist Prompt: Piston
      mask DialogControl cont_tensioner_brkt Prompt: Bracket
      mask DialogControl cont_tensioner_assy Prompt: Assembly
      mask DialogControl Container20 Prompt: Sensing
      mask Display: image('sm_excv_track_rollers_IMAGE.png');
  I : PMIOPort  Side=Right
  R : PMIOPort  Port=2  Side=Right
  Ref : PMIOPort  Port=3  Side=Right
  T : PMIOPort  Port=4  Side=Right
  Sh : PMIOPort  Port=5  Side=Right
  m : Outport
  wires:
  Rollers/1(m) -> m/1
  connections:
  Sh/RConn1 -- Rollers/RConn4
  Frame/RConn2 -- Rollers/LConn2
  Frame/RConn3 -- Rollers/LConn3
  Frame/RConn11 -- Rollers/LConn11
  Frame/RConn1 -- Rollers/LConn1
  Frame/RConn6 -- Rollers/LConn6
  Frame/RConn9 -- Rollers/LConn9
  Frame/RConn10 -- Rollers/LConn10
  Frame/RConn8 -- Rollers/LConn8
  Frame/RConn4 -- Rollers/LConn4
  Frame/RConn5 -- Rollers/LConn5
  Frame/RConn7 -- Rollers/LConn7
  Rollers/RConn3 -- T/RConn1
  Rollers/RConn1 -- I/RConn1
  Frame/LConn1 -- Ref/RConn1
  Rollers/RConn2 -- R/RConn1
